simulink model "FinalProjectSim"  (R2024b)
settings: Solver=VariableStepAuto  StartTime=0.0  StopTime=50  RelTol=1e-3
values from neighbouring files (symbols this model uses):
  A = [ ... (first row only)    [FinalProject.m]
  A_obs = A-L*C    [FinalProject.m]
  B = [ ... (first row only)    [FinalProject.m]
  B_obs = [B L]    [FinalProject.m]
  C = [ ... (first row only)    [FinalProject.m]
  C_obs = eye(5)    [FinalProject.m]
  F = inv(M)    [FinalProject.m]
  ref = [0 ; 10]    [FinalProject.m]
  ref2 = [10000 ;1]    [FinalProject.m]
  x0 = [ 30000;9500;5000;0.5;0.95]    [FinalProject.m]
undefined symbols (not defined in the file or in its folder): K, L
libraries: simulink x4
settings Model: Creator=izzycollins  LastModifiedBy=izzycollins

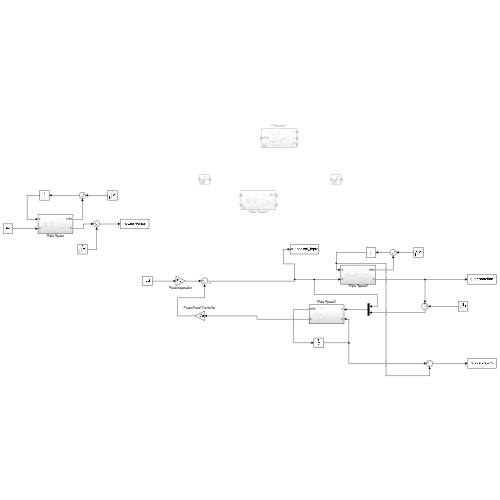
[thumbnail: Simulink's stored preview of the top-level diagram]
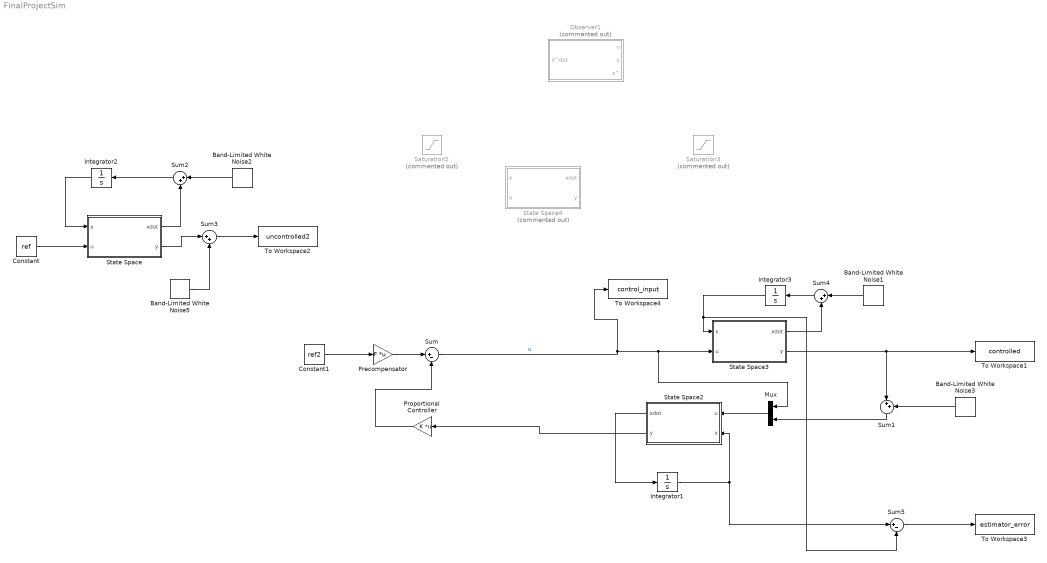
== system FinalProjectSim ==
  Band-Limited White Noise1 : simulink/Sources/Band-Limited White Noise  Cov=[1000;50;10;0.0002;0.0002]  Ts=1  seed=[23341]
  Band-Limited White Noise2 : simulink/Sources/Band-Limited White Noise  Cov=[1000;50;10;0.0002;0.0002]  Ts=1  seed=[23341]
  Band-Limited White Noise3 : simulink/Sources/Band-Limited White Noise  Cov=[1000;50;0.0002];  Ts=1  seed=[23341]
  Band-Limited White Noise5 : simulink/Sources/Band-Limited White Noise  Cov=[1000;50;0.0002];  Ts=1  seed=[23341]
  Constant : Constant  Value=ref
  Constant1 : Constant  Value=ref2
  Integrator1 : Integrator  InitialCondition=x0
  Integrator2 : Integrator  InitialCondition=x0
  Integrator3 : Integrator  InitialCondition=x0
  Mux : Mux  Inputs=2
  Observer1 : Subsystem  Commented=on
  Precompensator : Gain  Gain=F  Multiplication=Matrix(K*u)
  Proportional Controller : Gain  Gain=K  Multiplication=Matrix(K*u)
  Saturation2 : Saturate  Commented=on  UpperLimit=10000  LowerLimit=0
  Saturation3 : Saturate  Commented=on  UpperLimit=10000  LowerLimit=0
  State Space : Subsystem
  State Space2 : Subsystem
  State Space3 : Subsystem
  State Space4 : Subsystem  Commented=on
  Sum : Sum  Inputs=|+-
  Sum{1..4} (4 alike) : Sum  Inputs=|++
  Sum5 : Sum  Inputs=|+-
  To Workspace1 : ToWorkspace  VariableName=controlled  SaveFormat=Structure With Time  SampleTime=-1
  To Workspace2 : ToWorkspace  VariableName=uncontrolled2  SaveFormat=Structure With Time  SampleTime=-1
  To Workspace3 : ToWorkspace  VariableName=estimator_error  SaveFormat=Structure With Time  SampleTime=-1
  To Workspace4 : ToWorkspace  VariableName=control_input  SaveFormat=Structure With Time  SampleTime=-1
  wires:
  Constant/1 -> State Space/2(u)
  State Space2/1(xdot) -> Integrator1/1
  Proportional Controller/1 -> Sum/2
  Precompensator/1 -> Sum/1
  Constant1/1 -> Precompensator/1
  Integrator1/1 -> State Space2/2(x), Sum5/1
  State Space3/2(y) -> Sum1/1, To Workspace1/1
  Integrator2/1 -> State Space/1(x)
  State Space/1(xdot) -> Sum2/2
  Sum2/1 -> Integrator2/1
  State Space/2(y) -> Sum3/1
  Sum3/1 -> To Workspace2/1
  Band-Limited White Noise5/1 -> Sum3/2
  Band-Limited White Noise2/1 -> Sum2/1
  Band-Limited White Noise1/1 -> Sum4/1
  Sum4/1 -> Integrator3/1
  State Space3/1(xdot) -> Sum4/2
  Integrator3/1 -> Sum5/2, State Space3/1(x)
  Band-Limited White Noise3/1 -> Sum1/2
  Mux/1 -> State Space2/1(u)
  State Space2/2(y) -> Proportional Controller/1
  Sum1/1 -> Mux/2
  Sum5/1 -> To Workspace3/1
  Sum/1 -> To Workspace4/1, Mux/1, State Space3/2(u)  "u"

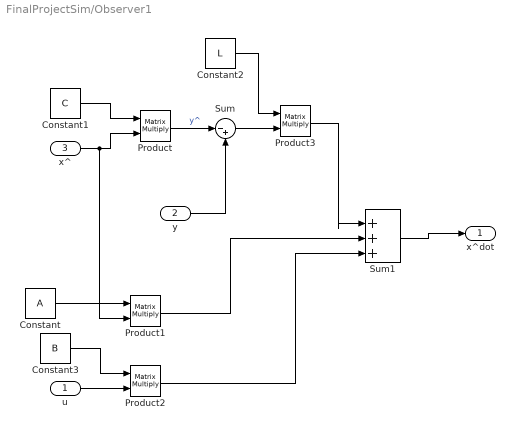
== system FinalProjectSim/Observer1 ==
  u : Inport
  y : Inport  Port=2
  x^ : Inport  Port=3
  Constant : Constant  Value=A
  Constant1 : Constant  Value=C
  Constant2 : Constant  Value=L
  Constant3 : Constant  Value=B
  Product{,1..3} (4 alike) : Product  Multiplication=Matrix(*)
  Sum : Sum  Inputs=|-+
  Sum1 : Sum  Inputs=|+++
  x^dot : Outport
  wires:
  Sum1/1 -> x^dot/1
  Product2/1 -> Sum1/3
  Product1/1 -> Sum1/2
  Product3/1 -> Sum1/1
  Sum/1 -> Product3/2
  Constant3/1 -> Product2/1
  u/1 -> Product2/2
  Constant/1 -> Product1/1
  y/1 -> Sum/2
  x^/1 -> Product/2, Product1/2
  Constant2/1 -> Product3/1
  Product/1 -> Sum/1  "y^"
  Constant1/1 -> Product/1

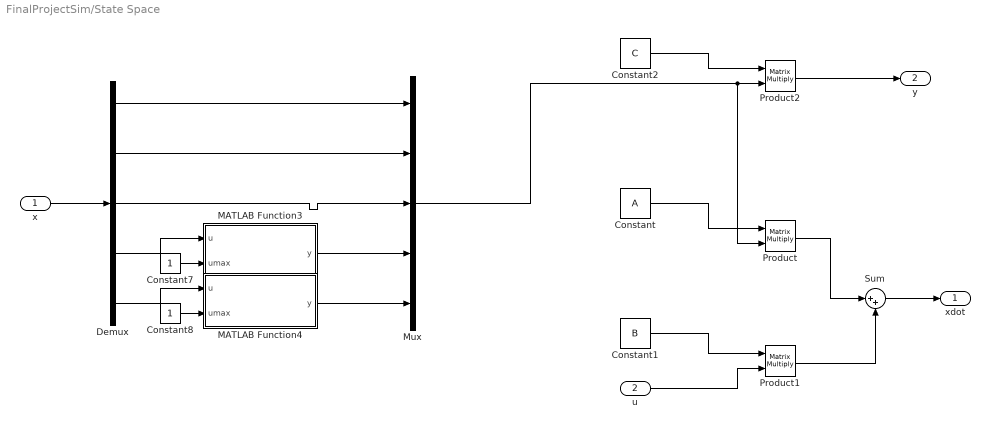
== system FinalProjectSim/State Space ==
  x : Inport
  u : Inport  Port=2
  Constant : Constant  Value=A
  Constant1 : Constant  Value=B
  Constant2 : Constant  Value=C
  Constant7 : Constant
  Constant8 : Constant
  Demux : Demux  Outputs=5
  MATLAB Function3 : MATLAB Function  TreatAsAtomicUnit=on
  MATLAB Function4 : MATLAB Function  TreatAsAtomicUnit=on
  Mux : Mux  Inputs=5
  Product : Product  Multiplication=Matrix(*)
  Product1 : Product  Multiplication=Matrix(*)
  Product2 : Product  Multiplication=Matrix(*)
  Sum : Sum  Inputs=|++
  xdot : Outport
  y : Outport  Port=2
  wires:
  Constant/1 -> Product/1
  Constant1/1 -> Product1/1
  u/1 -> Product1/2
  Product/1 -> Sum/1
  Product1/1 -> Sum/2
  Sum/1 -> xdot/1
  Constant2/1 -> Product2/1
  Product2/1 -> y/1
  Mux/1 -> Product/2, Product2/2
  x/1 -> Demux/1
  Demux/1 -> Mux/1
  Demux/2 -> Mux/2
  Demux/3 -> Mux/3
  Demux/4 -> MATLAB Function3/1(u)
  MATLAB Function3/1(y) -> Mux/4
  Demux/5 -> MATLAB Function4/1(u)
  MATLAB Function4/1(y) -> Mux/5
  Constant7/1 -> MATLAB Function3/2(umax)
  Constant8/1 -> MATLAB Function4/2(umax)

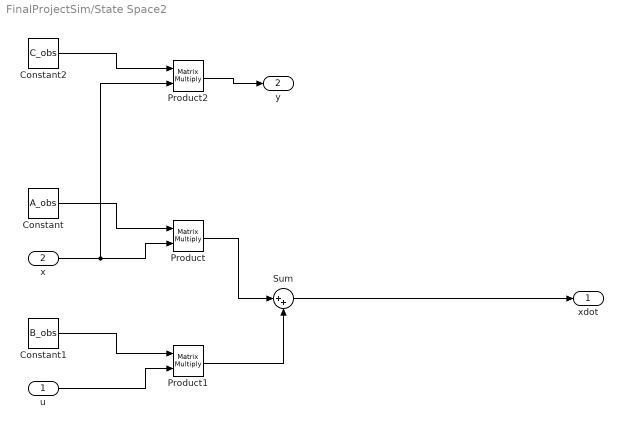
== system FinalProjectSim/State Space2 ==
  u : Inport
  x : Inport  Port=2
  Constant : Constant  Value=A_obs
  Constant1 : Constant  Value=B_obs
  Constant2 : Constant  Value=C_obs
  Product : Product  Multiplication=Matrix(*)
  Product1 : Product  Multiplication=Matrix(*)
  Product2 : Product  Multiplication=Matrix(*)
  Sum : Sum  Inputs=|++
  xdot : Outport
  y : Outport  Port=2
  wires:
  Constant/1 -> Product/1
  x/1 -> Product2/2, Product/2
  Constant1/1 -> Product1/1
  u/1 -> Product1/2
  Product/1 -> Sum/1
  Product1/1 -> Sum/2
  Sum/1 -> xdot/1
  Constant2/1 -> Product2/1
  Product2/1 -> y/1

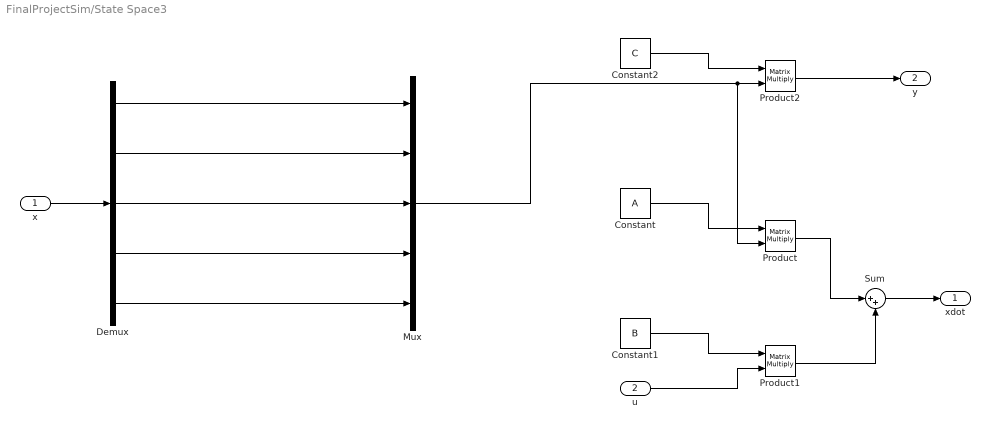
== system FinalProjectSim/State Space3 ==
  x : Inport
  u : Inport  Port=2
  Constant : Constant  Value=A
  Constant1 : Constant  Value=B
  Constant2 : Constant  Value=C
  Demux : Demux  Outputs=5
  Mux : Mux  Inputs=5
  Product : Product  Multiplication=Matrix(*)
  Product1 : Product  Multiplication=Matrix(*)
  Product2 : Product  Multiplication=Matrix(*)
  Sum : Sum  Inputs=|++
  xdot : Outport
  y : Outport  Port=2
  wires:
  Constant/1 -> Product/1
  Constant1/1 -> Product1/1
  u/1 -> Product1/2
  Product/1 -> Sum/1
  Product1/1 -> Sum/2
  Sum/1 -> xdot/1
  Constant2/1 -> Product2/1
  Product2/1 -> y/1
  Demux/5 -> Mux/5
  Demux/4 -> Mux/4
  Demux/3 -> Mux/3
  Demux/2 -> Mux/2
  Demux/1 -> Mux/1
  Mux/1 -> Product/2, Product2/2
  x/1 -> Demux/1

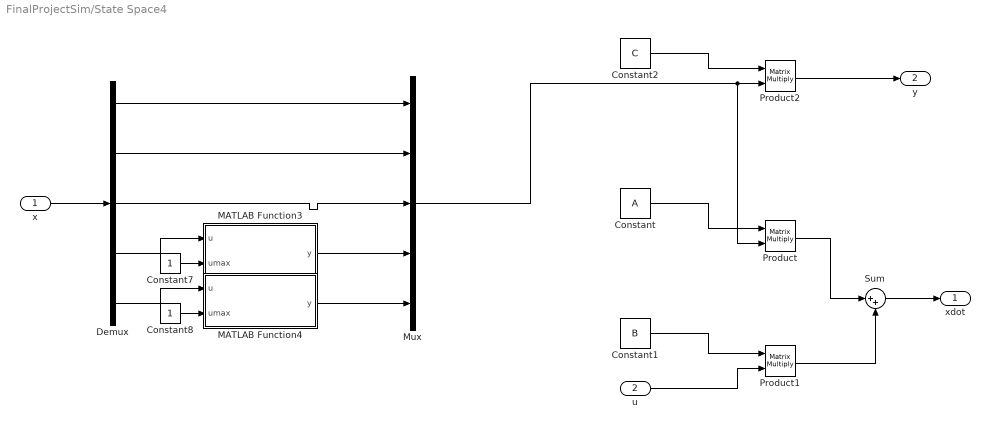
== system FinalProjectSim/State Space4 ==
  x : Inport
  u : Inport  Port=2
  Constant : Constant  Value=A
  Constant1 : Constant  Value=B
  Constant2 : Constant  Value=C
  Constant7 : Constant
  Constant8 : Constant
  Demux : Demux  Outputs=5
  MATLAB Function3 : MATLAB Function  TreatAsAtomicUnit=on
  MATLAB Function4 : MATLAB Function  TreatAsAtomicUnit=on
  Mux : Mux  Inputs=5
  Product : Product  Multiplication=Matrix(*)
  Product1 : Product  Multiplication=Matrix(*)
  Product2 : Product  Multiplication=Matrix(*)
  Sum : Sum  Inputs=|++
  xdot : Outport
  y : Outport  Port=2
  wires:
  Constant/1 -> Product/1
  Constant1/1 -> Product1/1
  u/1 -> Product1/2
  Product/1 -> Sum/1
  Product1/1 -> Sum/2
  Sum/1 -> xdot/1
  Constant2/1 -> Product2/1
  Product2/1 -> y/1
  Mux/1 -> Product/2, Product2/2
  x/1 -> Demux/1
  Demux/1 -> Mux/1
  Demux/2 -> Mux/2
  Demux/3 -> Mux/3
  Demux/4 -> MATLAB Function3/1(u)
  MATLAB Function3/1(y) -> Mux/4
  Demux/5 -> MATLAB Function4/1(u)
  MATLAB Function4/1(y) -> Mux/5
  Constant7/1 -> MATLAB Function3/2(umax)
  Constant8/1 -> MATLAB Function4/2(umax)

== matlab function FinalProjectSim/State Space4/MATLAB Function3 ==
  data: u input; y output; umax input
function y = smoothSat(u, umax)
% Smooth saturation using tanh
% u   = input
% umin, umax = lower/upper saturation limits
% k   = sharpness (typical values: 1 to 10)
umin = 0;
k = 5;
u_center = (umax + umin) / 2;
u_half   = (umax - umin) / 2;
y = u_center + u_half * tanh(k * (u - u_center) / u_half);
end

== matlab function FinalProjectSim/State Space/MATLAB Function3 ==
  data: u input; y output; umax input
function y = smoothSat(u, umax)
% Smooth saturation using tanh
% u   = input
% umin, umax = lower/upper saturation limits
% k   = sharpness (typical values: 1 to 10)
umin = 0;
k = 5;
u_center = (umax + umin) / 2;
u_half   = (umax - umin) / 2;
y = u_center + u_half * tanh(k * (u - u_center) / u_half);
end

== matlab function FinalProjectSim/State Space/MATLAB Function4 ==
  data: u input; y output; umax input
function y = smoothSat(u, umax)
% Smooth saturation using tanh
% u   = input
% umin, umax = lower/upper saturation limits
% k   = sharpness (typical values: 1 to 10)
umin = 0;
k = 5;
u_center = (umax + umin) / 2;
u_half   = (umax - umin) / 2;
y = u_center + u_half * tanh(k * (u - u_center) / u_half);
end

== matlab function FinalProjectSim/State Space4/MATLAB Function4 ==
  data: u input; y output; umax input
function y = smoothSat(u, umax)
% Smooth saturation using tanh
% u   = input
% umin, umax = lower/upper saturation limits
% k   = sharpness (typical values: 1 to 10)
umin = 0;
k = 5;
u_center = (umax + umin) / 2;
u_half   = (umax - umin) / 2;
y = u_center + u_half * tanh(k * (u - u_center) / u_half);
end
